simulink model "untitled"  (R2020a)
settings: Solver=VariableStepAuto  StartTime=0.0  StopTime=10.0  RelTol=1e-3
undefined symbols (not defined in the file or in its folder): f
libraries: instrumentlib x2
settings Model: Creator=assem  LastModifiedBy=assem

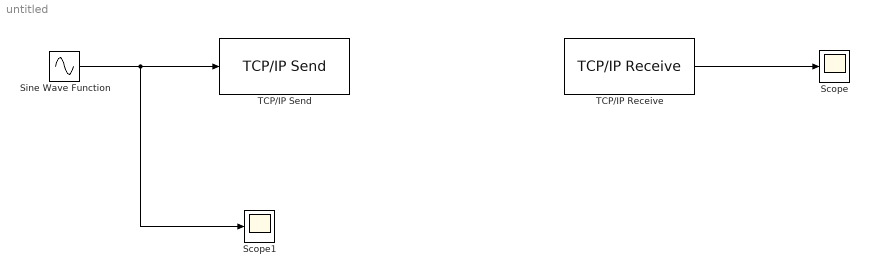
== system untitled ==
  Scope : Scope
  Scope1 : Scope
  Sine Wave Function : Sin  TimeSource=Use external signal  SampleTime=0
  TCP/IP Receive : instrumentlib/TCP//IP Receive  Host=127.0.0.1  Port=80  DataSize=[1 1]  EnableBlockingMode=on  Timeout=10  SampleTime=0.01  DataType=uint8  ByteOrder=BigEndian  ASCIIFormatting=%f,  Terminator=LF
  TCP/IP Send : instrumentlib/TCP//IP Send  Host=127.0.0.1  Port=80  EnableBlockingMode=on  Timeout=10  ByteOrder=BigEndian  TransferDelay=on
  wires:
  TCP/IP Receive/1 -> Scope/1
  Sine Wave Function/1 -> Scope1/1, TCP/IP Send/1
